simulink model "SAME5xPIM_MCLV2_MotorControl_Simulation"  (R2020b)
settings: Solver=ode45  StartTime=0.0  StopTime=10  FixedStep=0.001  MaxStep=1e-4  RelTol=1e-3  EnableMultiTasking=on
undefined symbols (not defined in the file or in its folder): DiscIntNeverNeededParam
libraries: simulink x8
Description:
  | Motor Control Simulation Demo
  | contacts : romain.delpoux@insa-lyon.fr, lubin.kerhuel@microchip.com
settings Model: DSRTSU_INTERNAL_RTI_VER=470  DSRTSU_INTERNAL_RTI_TYPE=rti1104  DSRTSU_INTERNAL_RTIFPGA=60  Creator=rdelpoux  LastModifiedBy=promu
settings SolverCC: ZeroCrossControl=DisableAll
settings DataIOCC: LimitDataPoints=on  SaveFormat=Array  ReturnWorkspaceOutputs=off
settings OptimizationCC: BlockReduction=off  OptimizeBlockIOStorage=off  BufferReuse=off  GlobalBufferReuse=off  ExpressionFolding=off  LocalBlockOutputs=off  LifeSpan=inf  OptimizeDataStoreBuffers=off  BusAssignmentInplaceUpdate=off
settings DebuggingCC: SolverPrmCheckMsg=warning  SFUnexpectedBacktrackingDiag=warning  SFNoUnconditionalDefaultTransitionDiag=warning  SFExecutionAtInitializationDiag=none  ArithmeticOperatorsInVariantConditions=warning
settings HardwareCC: ProdBitPerPointer=32  ProdBitPerSizeT=32  ProdBitPerPtrDiffT=32  ProdLargestAtomicInteger=Integer  ProdEndianess=BigEndian  ProdWordSize=32  ProdHWDeviceType=Generic->Custom  TargetIntDivRoundTo=Zero  TargetEndianess=BigEndian  TargetHWDeviceType=Generic->Custom
settings ModelReferenceCC: PropagateSignalLabelsOutOfModel=off
settings SFSimCC: SimUseLocalCustomCode=off  CustomCodeUndefinedFunction=UseInterfaceOnly
settings RTWCC: Description=dSPACE DS1104 Hardware Platform  SystemTargetFile=rti1104.tlc  MakeCommand=make_rti  TemplateMakefile=rti1104.tmf  RTWUseLocalCustomCode=off
settings CodeAppCC: StateflowObjectComments=on
settings STFCustomTargetCC: ParMdlRefBuildCompliant=on  ConcurrentExecutionCompliant=off  MatFileLogging=on  CPPClassGenCompliant=off  SystemTargetFile=rti1104.tlc
settings GRTTargetCC: TargetLangStandard=C89/C90 (ANSI)  CompOptLevelCompliant=off  ConcurrentExecutionCompliant=off  CombineOutputUpdateFcns=off  CPPClassGenCompliant=off  GRTInterface=on  UseToolchainInfoCompliant=off  ExtModeMexFile=noextcomm
settings ConfigComp: CovMetricSettings=dw  CovSaveCumulativeToWorkspaceVar=on  CovSaveSingleToWorkspaceVar=on  CovExternalEMLEnable=off  CovSFcnEnable=off

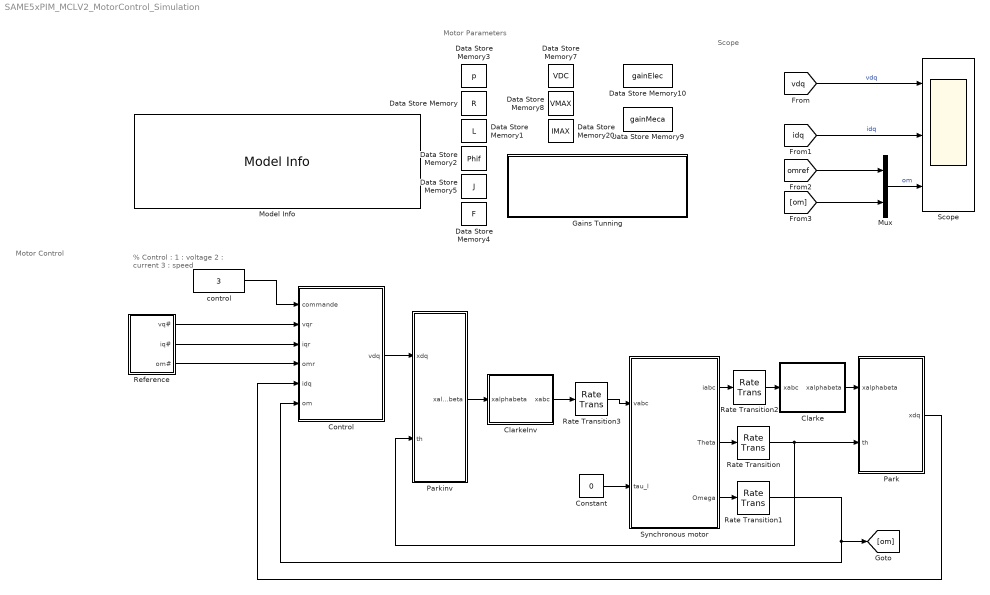
== system SAME5xPIM_MCLV2_MotorControl_Simulation ==
  note: Scope
  note: Motor Control
  note: % Control :
      | 1 : voltage
      | 2 : current
      | 3 : speed
  note: Motor Parameters
  Clarke : Subsystem
  ClarkeInv : Subsystem
  Constant : Constant  Value=0
  Control : Subsystem
  Data Store Memory : DataStoreMemory  DataStoreName=R  ReadBeforeWriteMsg=warning  WriteAfterWriteMsg=warning  WriteAfterReadMsg=warning  InitialValue=0.656  ShowAdditionalParam=off  OutDataTypeStr=single
  Data Store Memory1 : DataStoreMemory  DataStoreName=L  ReadBeforeWriteMsg=warning  WriteAfterWriteMsg=warning  WriteAfterReadMsg=warning  InitialValue=0.35e-3  ShowAdditionalParam=off  OutDataTypeStr=single
  Data Store Memory10 : DataStoreMemory  DataStoreName=gainElec  ReadBeforeWriteMsg=warning  WriteAfterWriteMsg=warning  WriteAfterReadMsg=warning  InitialValue=[0;0]  ShowAdditionalParam=off  OutDataTypeStr=single
  Data Store Memory2 : DataStoreMemory  DataStoreName=Phif  ReadBeforeWriteMsg=warning  WriteAfterWriteMsg=warning  WriteAfterReadMsg=warning  InitialValue=0.0066  ShowAdditionalParam=off  OutDataTypeStr=single
  Data Store Memory20 : DataStoreMemory  DataStoreName=IMAX  ReadBeforeWriteMsg=warning  WriteAfterWriteMsg=warning  WriteAfterReadMsg=warning  InitialValue=4  ShowAdditionalParam=off  OutDataTypeStr=int16
  Data Store Memory3 : DataStoreMemory  DataStoreName=p  ReadBeforeWriteMsg=warning  WriteAfterWriteMsg=warning  WriteAfterReadMsg=warning  InitialValue=4  ShowAdditionalParam=off  OutDataTypeStr=int16
  Data Store Memory4 : DataStoreMemory  DataStoreName=F  ReadBeforeWriteMsg=warning  WriteAfterWriteMsg=warning  WriteAfterReadMsg=warning  InitialValue=1.0e-05  ShowAdditionalParam=off  OutDataTypeStr=single
  Data Store Memory5 : DataStoreMemory  DataStoreName=J  ReadBeforeWriteMsg=warning  WriteAfterWriteMsg=warning  WriteAfterReadMsg=warning  InitialValue=1.0e-05  ShowAdditionalParam=off  OutDataTypeStr=single
  Data Store Memory7 : DataStoreMemory  DataStoreName=VDC  ReadBeforeWriteMsg=warning  WriteAfterWriteMsg=warning  WriteAfterReadMsg=warning  InitialValue=24  ShowAdditionalParam=off  OutMin=[-30]  OutMax=[30]  OutDataTypeStr=fixdt(1,16)
  Data Store Memory8 : DataStoreMemory  DataStoreName=VMAX  ReadBeforeWriteMsg=warning  WriteAfterWriteMsg=warning  WriteAfterReadMsg=warning  InitialValue=12  ShowAdditionalParam=off  OutMin=[-30]  OutMax=[30]  OutDataTypeStr=fixdt(1,16)
  Data Store Memory9 : DataStoreMemory  DataStoreName=gainMeca  ReadBeforeWriteMsg=warning  WriteAfterWriteMsg=warning  WriteAfterReadMsg=warning  InitialValue=[0;0]  ShowAdditionalParam=off  OutDataTypeStr=single
  Gains Tunning : Subsystem
  Model Info : simulink/Model-Wide Utilities/Model Info  Frame=on  DisplayStringWithTags=|  HorizontalTextAlignment=Center  LeftAlignmentValue=0.5
      | %<ModelName> v%<ModelVersion> - %<Creator>
      | 
      | %<Description>
      | 
      | Last modified on: %<LastModificationDate>
  Mux : Mux  Inputs=2
  "Park " : Subsystem
  Parkinv : Subsystem
  Rate Transition{,1..3} (4 alike) : RateTransition  OutPortSampleTime=1e-4
  Reference : Subsystem
  Scope : Scope  NumInputPorts=3
  Synchronous motor : Subsystem  mask(Test){Rmodel=0.656, Lmodel=0.35e-3, Phifmodel=0.0066, pmodel=4, Jmodel=1.e-05, fmodel=1.e-05, C0Model=0.01}
      mask prompts: Rmodel "Phase resistor R (Ohm)"; Lmodel "Phase Inductor L (H)"; Phifmodel "Rotor flux Phif (Wb)"; pmodel "Pole paires"; Jmodel "Inertia J (kg.m^2)"; fmodel "Fluide friction f (N.m.s/rad)"; C0Model "Dry friction C0 (N.m)"
      mask Help: disp('{\itEquation:}  \alpha^2 + \beta^2 \rightarrow \gamma^2, \chi, \phi_3 = {\bfcool}', 'texmode','on')
      mask DialogControl DescGroupVar Prompt: PMSM
      mask DialogControl DescTextVar Prompt: Motor Model
      mask DialogControl Container3 Prompt: Electrical parameters
      mask DialogControl Container4 Prompt: Mechanical parameter
  control : Constant  Value=3
  wires:
  Parkinv/1(xalphabeta) -> ClarkeInv/1(xalphabeta)
  ClarkeInv/1(xabc) -> Rate Transition3/1
  Rate Transition2/1 -> Clarke/1(xabc)
  Clarke/1(xalphabeta) -> "Park "/1(xalphabeta)
  "Park "/1(xdq) -> Control/5(idq)
  Reference/2(iq#) -> Control/3(iqr)
  Rate Transition1/1 -> [om], Control/6(om)
  Reference/3(om#) -> Control/4(omr)
  Rate Transition/1 -> Parkinv/2(th), "Park "/2(th)
  Control/1(vdq) -> Parkinv/1(xdq)
  Synchronous motor/3(Omega) -> Rate Transition1/1
  Synchronous motor/2(Theta) -> Rate Transition/1
  Synchronous motor/1(iabc) -> Rate Transition2/1
  Rate Transition3/1 -> Synchronous motor/1(vabc)
  control/1 -> Control/1(commande)
  Constant/1 -> Synchronous motor/2(tau_l)
  Reference/1(vq#) -> Control/2(vqr)
  [vdq] -> Scope/1  "vdq"
  [idq] -> Scope/2  "idq"
  [omref] -> Mux/1
  [om] -> Mux/2
  Mux/1 -> Scope/3  "om"

== system SAME5xPIM_MCLV2_MotorControl_Simulation/Clarke ==
  note: Clarke inverse
  xabc : Inport
  C23 : Gain  Gain=|  Multiplication=Matrix(K*u)
      | [1   -1/2        -1/2;
      |         0   sqrt(3)/2   -sqrt(3)/2]
  Gain : Gain  Gain=2/3
  xalphabeta : Outport  VectorParamsAs1DForOutWhenUnconnected=off
  wires:
  Gain/1 -> C23/1
  C23/1 -> xalphabeta/1
  xabc/1 -> Gain/1

== system SAME5xPIM_MCLV2_MotorControl_Simulation/ClarkeInv ==
  note: Clarke inverse
  xalphabeta : Inport
  C23' : Gain  Gain=|  Multiplication=Matrix(K*u)
      | [1   -1/2        -1/2;
      |         0   sqrt(3)/2   -sqrt(3)/2]'
  xabc : Outport  VectorParamsAs1DForOutWhenUnconnected=off
  wires:
  C23'/1 -> xabc/1
  xalphabeta/1 -> C23'/1

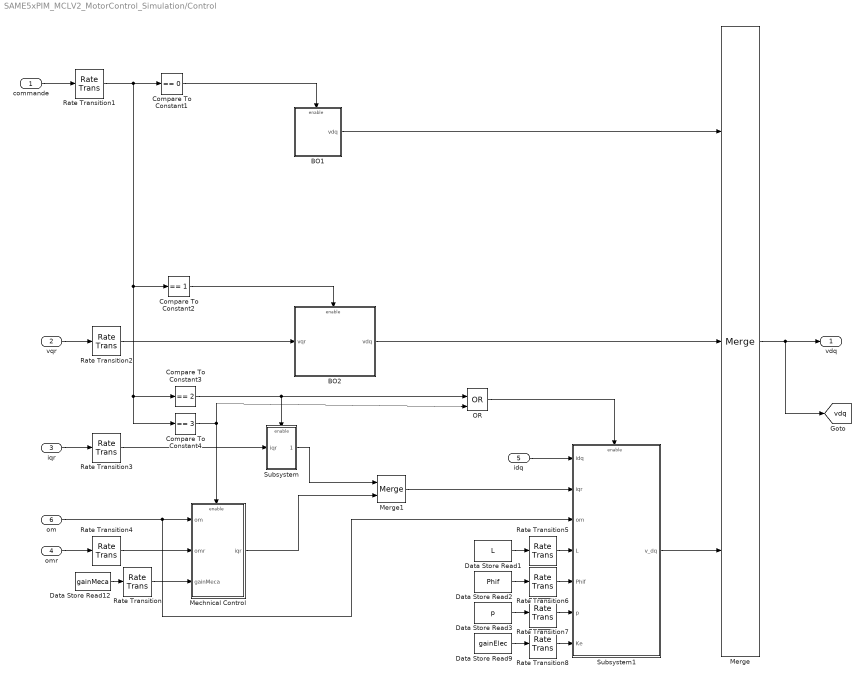
== system SAME5xPIM_MCLV2_MotorControl_Simulation/Control ==
  commande : Inport
  vqr : Inport  Port=2
  iqr : Inport  Port=3
  omr : Inport  Port=4
  idq : Inport  Port=5
  om : Inport  Port=6
  BO1 : Subsystem
  BO2 : Subsystem
  Compare To Constant1 : simulink/Logic and Bit Operations/Compare To Constant  relop===  const=0  OutDataTypeStr=boolean
  Compare To Constant2 : simulink/Logic and Bit Operations/Compare To Constant  relop===  const=1  OutDataTypeStr=boolean
  Compare To Constant3 : simulink/Logic and Bit Operations/Compare To Constant  relop===  const=2  OutDataTypeStr=boolean
  Compare To Constant4 : simulink/Logic and Bit Operations/Compare To Constant  relop===  const=3  OutDataTypeStr=boolean
  Data Store Read1 : DataStoreRead  DataStoreName=L  SampleTime=1
  Data Store Read12 : DataStoreRead  DataStoreName=gainMeca  SampleTime=1
  Data Store Read2 : DataStoreRead  DataStoreName=Phif  SampleTime=1
  Data Store Read3 : DataStoreRead  DataStoreName=p  SampleTime=1
  Data Store Read9 : DataStoreRead  DataStoreName=gainElec  SampleTime=1
  Mechnical Control : Subsystem
  Merge : Merge  Inputs=3
  Merge1 : Merge
  OR : Logic  Operator=OR  IconShape=distinctive  AllPortsSameDT=off  OutDataTypeStr=boolean
  Rate Transition{,1..8} (9 alike) : RateTransition
  Subsystem : Subsystem
  Subsystem1 : Subsystem
  vdq : Outport  VectorParamsAs1DForOutWhenUnconnected=off
  tag scope: vdq=global
  wires:
  Rate Transition8/1 -> Subsystem1/7(Ke)
  Rate Transition7/1 -> Subsystem1/6(p)
  Rate Transition6/1 -> Subsystem1/5(Phif)
  Rate Transition5/1 -> Subsystem1/4(L)
  Rate Transition/1 -> Mechnical Control/3(gainMeca)
  Rate Transition4/1 -> Mechnical Control/2(omr)
  Rate Transition3/1 -> Subsystem/1(iqr)
  Rate Transition2/1 -> BO2/1(vqr)
  Subsystem1/1(v_dq) -> Merge/3
  Merge1/1 -> Subsystem1/2(iqr)
  idq/1 -> Subsystem1/1(idq)
  OR/1 -> Subsystem1/Enable
  om/1 -> Mechnical Control/1(om), Subsystem1/3(om)
  Compare To Constant4/1 -> Mechnical Control/Enable, OR/2
  Mechnical Control/1(iqr) -> Merge1/2
  Subsystem/1(Out1) -> Merge1/1
  Rate Transition1/1 -> Compare To Constant1/1, Compare To Constant4/1, Compare To Constant3/1, Compare To Constant2/1
  Compare To Constant3/1 -> Subsystem/Enable, OR/1
  Compare To Constant1/1 -> BO1/Enable
  commande/1 -> Rate Transition1/1
  Merge/1 -> [vdq], vdq/1
  Compare To Constant2/1 -> BO2/Enable
  BO1/1(vdq) -> Merge/1
  BO2/1(vdq) -> Merge/2
  Data Store Read9/1 -> Rate Transition8/1
  Data Store Read1/1 -> Rate Transition5/1
  Data Store Read3/1 -> Rate Transition7/1
  Data Store Read2/1 -> Rate Transition6/1
  vqr/1 -> Rate Transition2/1
  iqr/1 -> Rate Transition3/1
  omr/1 -> Rate Transition4/1
  Data Store Read12/1 -> Rate Transition/1

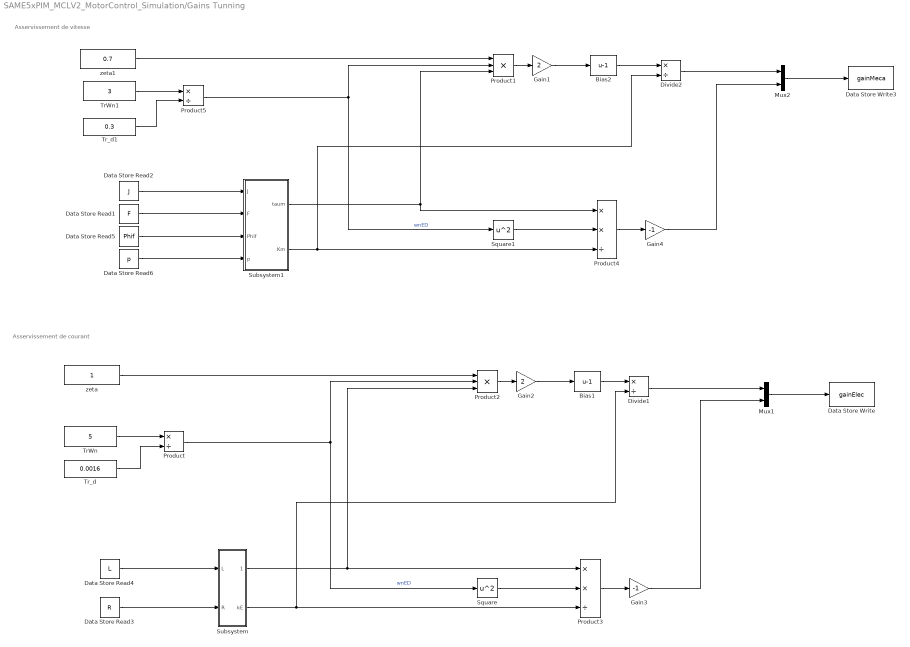
== system SAME5xPIM_MCLV2_MotorControl_Simulation/Gains Tunning ==
  note: Asservissement de courant
  note: Asservissement de vitesse
  Bias1 : Bias  Bias=-1
  Bias2 : Bias  Bias=-1
  Data Store Read1 : DataStoreRead  DataStoreName=F  SampleTime=1
  Data Store Read2 : DataStoreRead  DataStoreName=J  SampleTime=1
  Data Store Read3 : DataStoreRead  DataStoreName=R  SampleTime=1
  Data Store Read4 : DataStoreRead  DataStoreName=L  SampleTime=1
  Data Store Read5 : DataStoreRead  DataStoreName=Phif  SampleTime=1
  Data Store Read6 : DataStoreRead  DataStoreName=p  SampleTime=1
  Data Store Write : DataStoreWrite  DataStoreName=gainElec  SampleTime=1
  Data Store Write3 : DataStoreWrite  DataStoreName=gainMeca
  Divide1 : Product  Inputs=*/
  Divide2 : Product  Inputs=*/
  Gain1 : Gain  Gain=2
  Gain2 : Gain  Gain=2
  Gain3 : Gain  Gain=-1
  Gain4 : Gain  Gain=-1
  Mux1 : Mux  Inputs=2
  Mux2 : Mux  Inputs=2
  Product : Product  Inputs=*/
  Product1 : Product  Inputs=3
  Product2 : Product  Inputs=3
  Product3 : Product  Inputs=**/
  Product4 : Product  Inputs=**/
  Product5 : Product  Inputs=*/
  Square : Math  Operator=square  SaturateOnIntegerOverflow=on
  Square1 : Math  Operator=square  SaturateOnIntegerOverflow=on
  Subsystem : Subsystem
  Subsystem1 : Subsystem
  TrWn : Constant  Value=5  OutDataTypeStr=single
  TrWn1 : Constant  Value=3  OutDataTypeStr=single
  Tr_d : Constant  Value=0.0016  OutDataTypeStr=single
  Tr_d1 : Constant  Value=0.3  OutDataTypeStr=single
  zeta : Constant  OutDataTypeStr=single
  zeta1 : Constant  Value=0.7  OutDataTypeStr=single
  wires:
  Gain3/1 -> Mux1/2
  Product3/1 -> Gain3/1
  Divide1/1 -> Mux1/1
  Bias1/1 -> Divide1/1
  Product2/1 -> Gain2/1
  Mux1/1 -> Data Store Write/1
  Data Store Read4/1 -> Subsystem/1(L)
  Data Store Read3/1 -> Subsystem/2(R)
  Subsystem/1(tauE) -> Product2/3, Product3/1
  TrWn/1 -> Product/1
  Tr_d/1 -> Product/2
  Product/1 -> Product2/2, Square/1  "wnED"
  Subsystem/2(kE) -> Divide1/2, Product3/3
  Gain2/1 -> Bias1/1
  zeta/1 -> Product2/1
  Square/1 -> Product3/2
  Square1/1 -> Product4/2
  Gain1/1 -> Bias2/1
  Product1/1 -> Gain1/1
  Bias2/1 -> Divide2/1
  Divide2/1 -> Mux2/1
  Product4/1 -> Gain4/1
  Gain4/1 -> Mux2/2
  Mux2/1 -> Data Store Write3/1
  Data Store Read2/1 -> Subsystem1/1(J)
  Data Store Read1/1 -> Subsystem1/2(F)
  Data Store Read5/1 -> Subsystem1/3(Phif)
  Data Store Read6/1 -> Subsystem1/4(p)
  Tr_d1/1 -> Product5/2
  TrWn1/1 -> Product5/1
  zeta1/1 -> Product1/1
  Product5/1 -> Square1/1, Product1/2  "wnED"
  Subsystem1/1(taum) -> Product4/1, Product1/3
  Subsystem1/2(Km) -> Divide2/2, Product4/3

== system SAME5xPIM_MCLV2_MotorControl_Simulation/Park  ==
  note: Inverse Park
  xalphabeta : Inport
  th : Inport  Port=2
  Fcn : Fcn  Expr=u(1)*cos(4*u(3))+u(2)*sin(4*u(3))
  Fcn1 : Fcn  Expr=-u(1)*sin(4*u(3))+u(2)*cos(4*u(3))
  Mux : Mux  Inputs=2
  Mux1 : Mux  Inputs=2
  xdq : Outport  VectorParamsAs1DForOutWhenUnconnected=off
  tag scope: idq=global
  wires:
  xalphabeta/1 -> Mux/1
  th/1 -> Mux/2
  Mux/1 -> Fcn1/1, Fcn/1
  Fcn/1 -> Mux1/1
  Fcn1/1 -> Mux1/2
  Mux1/1 -> [idq], xdq/1

== system SAME5xPIM_MCLV2_MotorControl_Simulation/Parkinv ==
  note: Inverse Park
  xdq : Inport
  th : Inport  Port=2
  Fcn : Fcn  Expr=u(1)*cos(4*u(3))-u(2)*sin(4*u(3))
  Fcn1 : Fcn  Expr=u(1)*sin(4*u(3))+u(2)*cos(4*u(3))
  Mux : Mux  Inputs=2
  Mux1 : Mux  Inputs=2
  xalphabeta : Outport  VectorParamsAs1DForOutWhenUnconnected=off
  wires:
  Mux1/1 -> xalphabeta/1
  Fcn1/1 -> Mux1/2
  Fcn/1 -> Mux1/1
  Mux/1 -> Fcn/1, Fcn1/1
  th/1 -> Mux/2
  xdq/1 -> Mux/1

== system SAME5xPIM_MCLV2_MotorControl_Simulation/Reference ==
  Step : Step  Time=2  After=2  OutDataTypeStr=single  SampleTime=0
  Step1 : Step  Time=2  After=300  OutDataTypeStr=single  SampleTime=0
  Step2 : Step  Time=2  After=5  OutDataTypeStr=single  SampleTime=0
  vq# : Outport  VectorParamsAs1DForOutWhenUnconnected=off
  iq# : Outport  Port=2  VectorParamsAs1DForOutWhenUnconnected=off
  om# : Outport  Port=3  VectorParamsAs1DForOutWhenUnconnected=off
  tag scope: omref=global
  wires:
  Step/1 -> iq#/1
  Step1/1 -> [omref], om#/1
  Step2/1 -> vq#/1

== system SAME5xPIM_MCLV2_MotorControl_Simulation/Synchronous motor ==
  vabc : Inport
  tau_l : Inport  Port=2
  Data Type Conversion : DataTypeConversion  OutDataTypeStr=single
  Data Type Conversion1 : DataTypeConversion  OutDataTypeStr=single
  Data Type Conversion2 : DataTypeConversion  OutDataTypeStr=single
  Electrique : Subsystem
  Mécanique : Subsystem
  iabc : Outport  VectorParamsAs1DForOutWhenUnconnected=off
  Theta : Outport  Port=2  VectorParamsAs1DForOutWhenUnconnected=off
  Omega : Outport  Port=3  VectorParamsAs1DForOutWhenUnconnected=off
  wires:
  vabc/1 -> Electrique/1(vabc)
  tau_l/1 -> Mécanique/2(tau_l)
  Electrique/1(iabc) -> Data Type Conversion/1
  Mécanique/1(Theta) -> Electrique/3(Theta), Data Type Conversion1/1
  Mécanique/2(Omega) -> Electrique/2(Omega), Data Type Conversion2/1
  Electrique/2(tau_m) -> Mécanique/1(tau_m)
  Data Type Conversion/1 -> iabc/1
  Data Type Conversion1/1 -> Theta/1
  Data Type Conversion2/1 -> Omega/1

== system SAME5xPIM_MCLV2_MotorControl_Simulation/Control/BO1 ==
  Enable : EnablePort
  Mux : Mux  Inputs=2
  vd : Constant  Value=0  OutMin=[-12]  OutMax=[12]  OutDataTypeStr=single
  vq : Constant  Value=0  OutMin=[-12]  OutMax=[12]  OutDataTypeStr=single
  vdq : Outport  VectorParamsAs1DForOutWhenUnconnected=off
  wires:
  vd/1 -> Mux/1
  Mux/1 -> vdq/1
  vq/1 -> Mux/2

== system SAME5xPIM_MCLV2_MotorControl_Simulation/Control/BO2 ==
  vqr : Inport
  Enable : EnablePort
  Constant : Constant  Value=0  OutDataTypeStr=single
  Mux : Mux  Inputs=2
  vdq : Outport  VectorParamsAs1DForOutWhenUnconnected=off
  wires:
  vqr/1 -> Mux/2
  Constant/1 -> Mux/1
  Mux/1 -> vdq/1

== system SAME5xPIM_MCLV2_MotorControl_Simulation/Control/Mechnical Control ==
  om : Inport
  omr : Inport  Port=2
  gainMeca : Inport  Port=3
  Enable : EnablePort  StatesWhenEnabling=reset
  Augmented state feedback : Subsystem
      settings: PortSchema="{\"entries\":[{\"content\":{\"sides\":[{\"content\":{\"connectorIds\":[\"In1\",\"In2\"]},\"type\":\"ConnectorPlacement.EquallySpacedRectSide\",\"uuid\":\"89137e2f-cd18-4dcc-a524-9caf5367be1f\"},{\"content\":{\"connectorIds\":[\"Out1\"],\"side\":\"RIGHT\"},\"type\":\"ConnectorPlacement.EquallySpacedRectSide\",\"uuid\":\"4fa0fb61-d5d6-47b2-9e74-7b8a54a26f7d\"},{\"content\":{\"connectorIds\":[],\"side\":\"TOP\"},\"type\":\"ConnectorPlacement.EquallySpacedRectSide\",\"uuid\":\"143a26d0-3cb3-43f1-872c-87316c90bc9f\"},{\"content\":{\"connectorIds\":[\"In3\"],\"side\":\"BOTTOM\"},\"type\":\"ConnectorPlacement.EquallySpacedRectSide\",\"uuid\":\"8516086b-4f00-45b1-b860-126256ccf69b\"},{\"content\":{\"connectorIds\":[],\"side\":\"HIDDEN\"},\"type\":\"ConnectorPlacement.EquallySpacedRectSide\",\"uuid\":\"abbfb321-16c4-4def-9c9f-eddb440e6971\"}]},\"type\":\"ConnectorPlacement.EquallySpacedConnector\",\"uuid\":\"ad3527e6-0bb9-4e51-b689-1365c7b23b5d\"}],\"packageUris\":[\"http://schema.mathworks.com/mf0/Connector/R2020b\"],\"version\":\"1.0\"}"
  iqr : Outport  VectorParamsAs1DForOutWhenUnconnected=off
  wires:
  om/1 -> Augmented state feedback/2(om)
  Augmented state feedback/1(iqref) -> iqr/1
  omr/1 -> Augmented state feedback/1(omref)
  gainMeca/1 -> Augmented state feedback/3(gainMeca)

== system SAME5xPIM_MCLV2_MotorControl_Simulation/Control/Subsystem ==
  iqr : Inport
  Enable : EnablePort
  Out1 : Outport
  wires:
  iqr/1 -> Out1/1

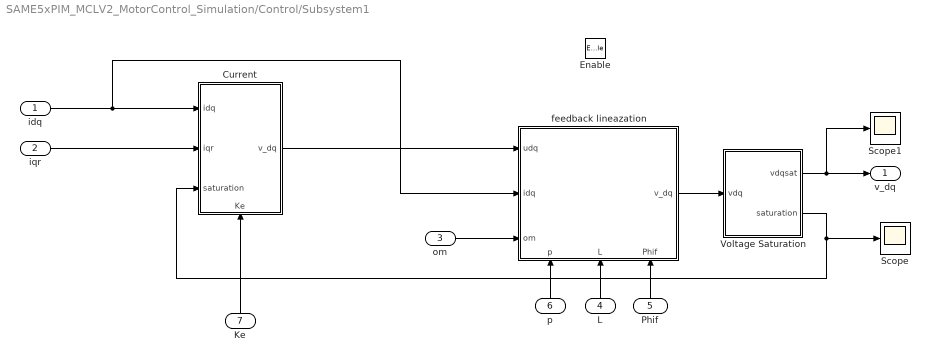
== system SAME5xPIM_MCLV2_MotorControl_Simulation/Control/Subsystem1 ==
  idq : Inport
  iqr : Inport  Port=2
  om : Inport  Port=3
  L : Inport  Port=4
  Phif : Inport  Port=5
  p : Inport  Port=6
  Ke : Inport  Port=7
  Enable : EnablePort  StatesWhenEnabling=reset
  Current : Subsystem
      settings: PortSchema="{\"entries\":[{\"content\":{\"sides\":[{\"content\":{\"connectorIds\":[\"In1\",\"In2\",\"In3\"]},\"type\":\"ConnectorPlacement.EquallySpacedRectSide\",\"uuid\":\"0dd1bd5c-4f2d-4a51-9bc2-8bf74640d4ff\"},{\"content\":{\"connectorIds\":[\"Out1\"],\"side\":\"RIGHT\"},\"type\":\"ConnectorPlacement.EquallySpacedRectSide\",\"uuid\":\"9ff54608-efe8-47a2-97c0-1c2807ae0451\"},{\"content\":{\"connectorIds\":[],\"side\":\"TOP\"},\"type\":\"ConnectorPlacement.EquallySpacedRectSide\",\"uuid\":\"a5b0a1bc-2629-443b-a6ad-4c332df72e2c\"},{\"content\":{\"connectorIds\":[\"In4\"],\"side\":\"BOTTOM\"},\"type\":\"ConnectorPlacement.EquallySpacedRectSide\",\"uuid\":\"e8d63822-9705-4716-821c-9412f2966827\"},{\"content\":{\"connectorIds\":[],\"side\":\"HIDDEN\"},\"type\":\"ConnectorPlacement.EquallySpacedRectSide\",\"uuid\":\"63401b5c-75e9-49e9-aa08-12658d9987d3\"}]},\"type\":\"ConnectorPlacement.EquallySpacedConnector\",\"uuid\":\"d3f45542-3ea7-483a-a2ee-6c72d9ae8820\"}],\"packageUris\":[\"http://schema.mathworks.com/mf0/Connector/R2020b\"],\"version\":\"1.0\"}"
  Scope : Scope
  Scope1 : Scope
  Voltage Saturation : Subsystem
  feedback lineazation : Subsystem
      settings: PortSchema="{\"entries\":[{\"content\":{\"sides\":[{\"content\":{\"connectorIds\":[\"In1\",\"In2\",\"In3\"]},\"type\":\"ConnectorPlacement.EquallySpacedRectSide\",\"uuid\":\"169b5321-ee7c-423e-8449-192a786c9798\"},{\"content\":{\"connectorIds\":[\"Out1\"],\"side\":\"RIGHT\"},\"type\":\"ConnectorPlacement.EquallySpacedRectSide\",\"uuid\":\"910fdd05-0903-4759-8f85-a6669ffcf15d\"},{\"content\":{\"connectorIds\":[],\"side\":\"TOP\"},\"type\":\"ConnectorPlacement.EquallySpacedRectSide\",\"uuid\":\"8e0cf6ac-18cd-4e02-9312-1598b8dbe459\"},{\"content\":{\"connectorIds\":[\"In4\",\"In5\",\"In6\"],\"side\":\"BOTTOM\"},\"type\":\"ConnectorPlacement.EquallySpacedRectSide\",\"uuid\":\"bf7c0436-036d-4f64-97d8-e9b131650054\"},{\"content\":{\"connectorIds\":[],\"side\":\"HIDDEN\"},\"type\":\"ConnectorPlacement.EquallySpacedRectSide\",\"uuid\":\"cd87405f-25ee-425b-a181-6989070156fa\"}]},\"type\":\"ConnectorPlacement.EquallySpacedConnector\",\"uuid\":\"912b1b6f-c896-42c8-9325-248c15d73689\"}],\"packageUris\":[\"http://schema.mathworks.com/mf0/Connector/R2020b\"],\"version\":\"1.0\"}"
  v_dq : Outport
  wires:
  om/1 -> feedback lineazation/3(om)
  L/1 -> feedback lineazation/5(L)
  Phif/1 -> feedback lineazation/6(Phif)
  p/1 -> feedback lineazation/4(p)
  Voltage Saturation/1(vdqsat) -> Scope1/1, v_dq/1
  iqr/1 -> Current/2(iqr)
  Current/1(v_dq) -> feedback lineazation/1(udq)
  idq/1 -> feedback lineazation/2(idq), Current/1(idq)
  Ke/1 -> Current/4(Ke)
  Voltage Saturation/2(saturation) -> Scope/1, Current/3(saturation)
  feedback lineazation/1(v_dq) -> Voltage Saturation/1(vdq)

== system SAME5xPIM_MCLV2_MotorControl_Simulation/Gains Tunning/Subsystem ==
  L : Inport
  R : Inport  Port=2
  Divide1 : Product  Inputs=/
  Divide2 : Product  Inputs=*/
  tauE : Outport
  kE : Outport  Port=2
  wires:
  Divide2/1 -> tauE/1  "tauE"
  R/1 -> Divide1/1, Divide2/2
  L/1 -> Divide2/1
  Divide1/1 -> kE/1  "kE"

== system SAME5xPIM_MCLV2_MotorControl_Simulation/Gains Tunning/Subsystem1 ==
  J : Inport
  F : Inport  Port=2
  Phif : Inport  Port=3
  p : Inport  Port=4
  Divide3 : Product  Inputs=*/
  Divide6 : Product  Inputs=*/
  Divide7 : Product  Inputs=**
  Gain : Gain  Gain=3/2
  taum : Outport
  Km : Outport  Port=2
  wires:
  Gain/1 -> Divide7/1
  F/1 -> Divide3/2, Divide6/2
  J/1 -> Divide6/1
  p/1 -> Divide7/2
  Divide3/1 -> Km/1  "Km"
  Phif/1 -> Gain/1
  Divide6/1 -> taum/1  "taum"
  Divide7/1 -> Divide3/1  "Km"

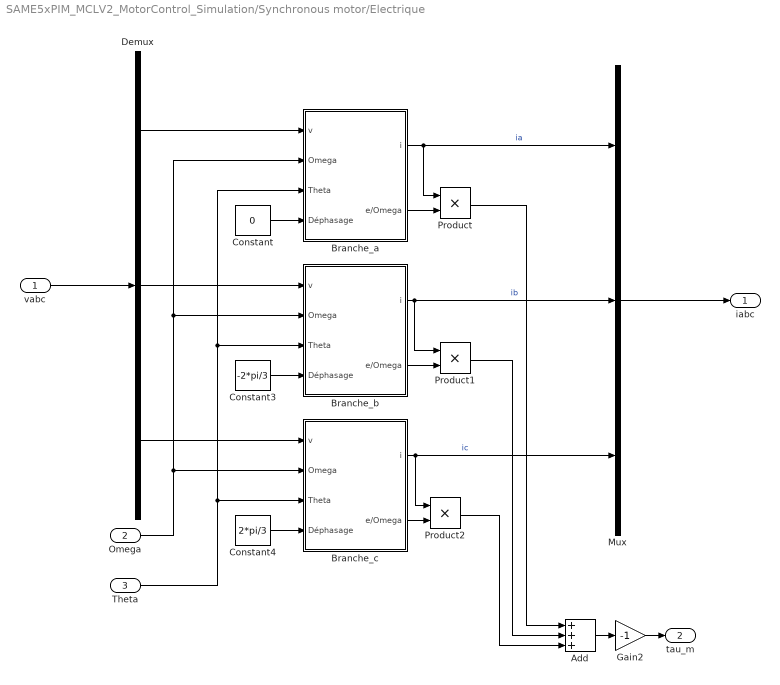
== system SAME5xPIM_MCLV2_MotorControl_Simulation/Synchronous motor/Electrique ==
  vabc : Inport
  Omega : Inport  Port=2
  Theta : Inport  Port=3
  Add : Sum  Inputs=+++
  Branche_a : Subsystem
  Branche_b : Subsystem
  Branche_c : Subsystem
  Constant : Constant  Value=0
  Constant3 : Constant  Value=-2*pi/3
  Constant4 : Constant  Value=2*pi/3
  Demux : Demux  Outputs=3
  Gain2 : Gain  Gain=-1
  Mux : Mux  Inputs=3
  Product : Product
  Product1 : Product
  Product2 : Product
  iabc : Outport  VectorParamsAs1DForOutWhenUnconnected=off
  tau_m : Outport  Port=2  VectorParamsAs1DForOutWhenUnconnected=off
  wires:
  Branche_c/1(i) -> Product2/1, Mux/3  "ic"
  Demux/1 -> Branche_a/1(v)
  Demux/2 -> Branche_b/1(v)
  Constant/1 -> Branche_a/4(Déphasage)
  Constant3/1 -> Branche_b/4(Déphasage)
  Constant4/1 -> Branche_c/4(Déphasage)
  Branche_b/1(i) -> Mux/2, Product1/1  "ib"
  Branche_a/1(i) -> Mux/1, Product/1  "ia"
  Demux/3 -> Branche_c/1(v)
  Theta/1 -> Branche_a/3(Theta), Branche_b/3(Theta), Branche_c/3(Theta)
  Omega/1 -> Branche_a/2(Omega), Branche_b/2(Omega), Branche_c/2(Omega)
  Branche_a/2(e/Omega) -> Product/2
  Branche_b/2(e/Omega) -> Product1/2
  Branche_c/2(e/Omega) -> Product2/2
  Product2/1 -> Add/3
  Product1/1 -> Add/2
  Product/1 -> Add/1
  Add/1 -> Gain2/1
  Gain2/1 -> tau_m/1
  Mux/1 -> iabc/1
  vabc/1 -> Demux/1

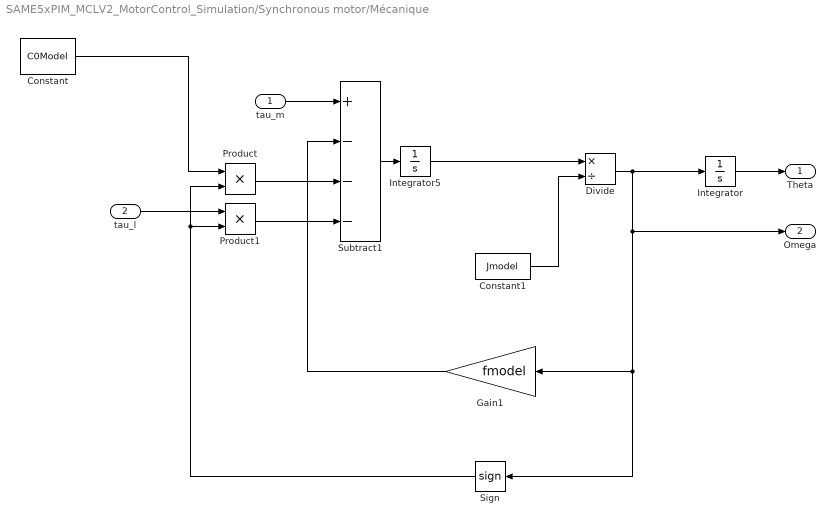
== system SAME5xPIM_MCLV2_MotorControl_Simulation/Synchronous motor/Mécanique ==
  tau_m : Inport
  tau_l : Inport  Port=2
  Constant : Constant  Value=C0Model
  Constant1 : Constant  Value=Jmodel
  Divide : Product  Inputs=*/
  Gain1 : Gain  Gain=fmodel
  Integrator : Integrator
  Integrator5 : Integrator
  Product : Product
  Product1 : Product
  Sign : Signum  ZeroCross=off
  Subtract1 : Sum  Inputs=+---
  Theta : Outport  VectorParamsAs1DForOutWhenUnconnected=off
  Omega : Outport  Port=2  VectorParamsAs1DForOutWhenUnconnected=off
  wires:
  Product/1 -> Subtract1/3
  Sign/1 -> Product1/2, Product/2
  Constant1/1 -> Divide/2
  Constant/1 -> Product/1
  tau_m/1 -> Subtract1/1
  Gain1/1 -> Subtract1/2
  Divide/1 -> Integrator/1, Omega/1, Gain1/1, Sign/1
  Integrator5/1 -> Divide/1
  tau_l/1 -> Product1/1
  Integrator/1 -> Theta/1
  Subtract1/1 -> Integrator5/1
  Product1/1 -> Subtract1/4

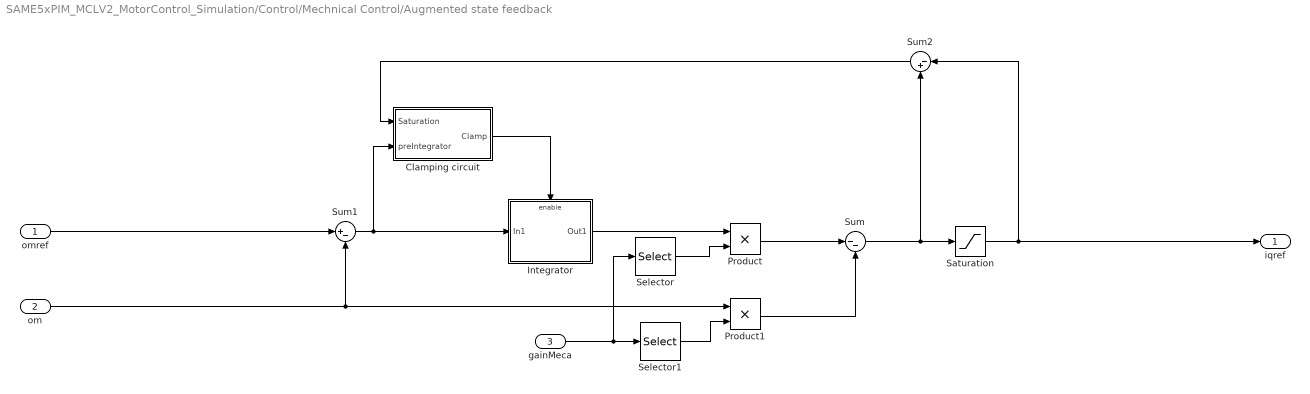
== system SAME5xPIM_MCLV2_MotorControl_Simulation/Control/Mechnical Control/Augmented state feedback ==
  omref : Inport
  om : Inport  Port=2
  gainMeca : Inport  Port=3
  Clamping circuit : Subsystem
  Integrator : Subsystem
  Product : Product
  Product1 : Product
  Saturation : Saturate  UpperLimit=4  LowerLimit=-4
  Selector : Selector  InputPortWidth=2  IndexOptions=Index vector (dialog)  Indices=[2]  OutputSizes=1
  Selector1 : Selector  InputPortWidth=2  IndexOptions=Index vector (dialog)  Indices=1  OutputSizes=1
  Sum : Sum  Inputs=|--  OutDataTypeStr=single  SaturateOnIntegerOverflow=on
  Sum1 : Sum  Inputs=|+-
  Sum2 : Sum  Inputs=|-+  OutDataTypeStr=Inherit: Same as accumulator  SaturateOnIntegerOverflow=on
  iqref : Outport  VectorParamsAs1DForOutWhenUnconnected=off
  wires:
  Sum/1 -> Sum2/2, Saturation/1
  Product1/1 -> Sum/2
  Product/1 -> Sum/1
  om/1 -> Sum1/2, Product1/1
  Sum1/1 -> Integrator/1(In1), Clamping circuit/2(preIntegrator)
  omref/1 -> Sum1/1
  Clamping circuit/1(Clamp) -> Integrator/Enable
  Sum2/1 -> Clamping circuit/1(Saturation)
  Integrator/1(Out1) -> Product/1
  Saturation/1 -> Sum2/1, iqref/1
  Selector1/1 -> Product1/2
  Selector/1 -> Product/2
  gainMeca/1 -> Selector1/1, Selector/1

== system SAME5xPIM_MCLV2_MotorControl_Simulation/Control/Subsystem1/Current ==
  idq : Inport
  iqr : Inport  Port=2
  saturation : Inport  Port=3
  Ke : Inport  Port=4
  Constant : Constant  Value=0
  Delay : Delay  DelayLength=1
  Gain1 : Gain  Gain=[1 0]  Multiplication=Matrix(K*u)  OutDataTypeStr=Inherit: Same as input
  Gain2 : Gain  Gain=[0 1]  Multiplication=Matrix(K*u)  OutDataTypeStr=Inherit: Same as input
  Gain3 : Gain  Gain=[1 0]  Multiplication=Matrix(K*u)  OutDataTypeStr=Inherit: Same as input
  Gain4 : Gain  Gain=[0 1]  Multiplication=Matrix(K*u)  OutDataTypeStr=Inherit: Same as input
  Mux1 : Mux  Inputs=2
  Subsystem1 : Subsystem
  Subsystem2 : Subsystem
  v_dq : Outport  VectorParamsAs1DForOutWhenUnconnected=off
  wires:
  Constant/1 -> Subsystem1/1(iref)
  saturation/1 -> Delay/1
  Subsystem2/1(v) -> Mux1/2
  Subsystem1/1(v) -> Mux1/1
  idq/1 -> Gain2/1, Gain1/1
  Gain1/1 -> Subsystem1/2(i)
  Gain2/1 -> Subsystem2/2(i)
  Mux1/1 -> v_dq/1
  Ke/1 -> Subsystem1/4(K_e), Subsystem2/4(K_e)
  Delay/1 -> Gain3/1, Gain4/1
  Gain3/1 -> Subsystem1/3(saturation)
  Gain4/1 -> Subsystem2/3(saturation)
  iqr/1 -> Subsystem2/1(iref)

== system SAME5xPIM_MCLV2_MotorControl_Simulation/Control/Subsystem1/Voltage Saturation ==
  vdq : Inport
  Divide : Product  Inputs=*/
  Gain : Gain  Gain=12
  Norm L2 : Subsystem
  Sum : Sum  Inputs=|+-
  Switch : Switch  Criteria=u2 > Threshold  Threshold=12
  vdqsat : Outport  VectorParamsAs1DForOutWhenUnconnected=off
  saturation : Outport  Port=2  VectorParamsAs1DForOutWhenUnconnected=off
  wires:
  Sum/1 -> saturation/1
  vdq/1 -> Switch/3, Sum/1, Divide/1, Norm L2/1(In1)
  Switch/1 -> vdqsat/1, Sum/2
  Divide/1 -> Gain/1
  Norm L2/1(y) -> Switch/2, Divide/2
  Gain/1 -> Switch/1

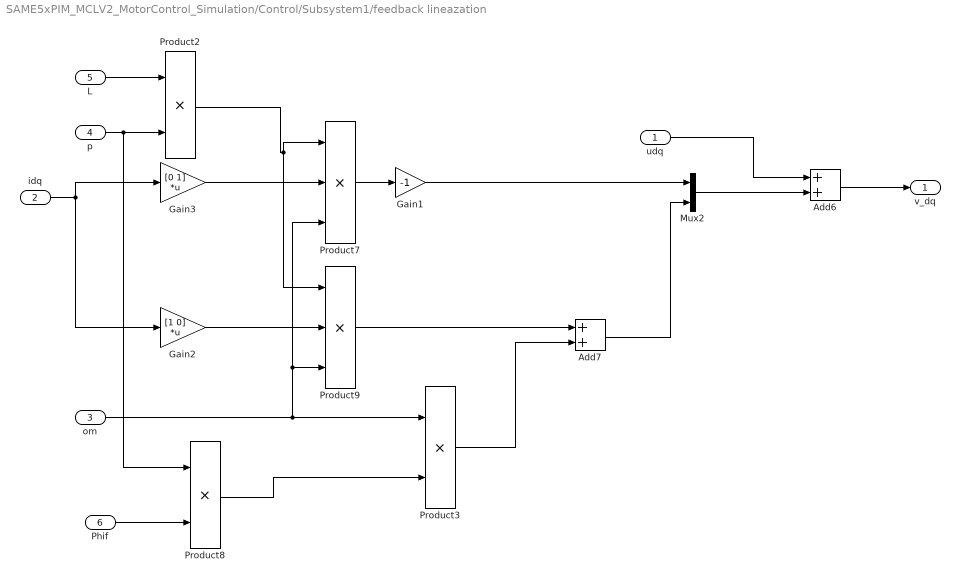
== system SAME5xPIM_MCLV2_MotorControl_Simulation/Control/Subsystem1/feedback lineazation ==
  udq : Inport
  idq : Inport  Port=2
  om : Inport  Port=3
  p : Inport  Port=4
  L : Inport  Port=5
  Phif : Inport  Port=6
  Add6 : Sum
  Add7 : Sum
  Gain1 : Gain  Gain=-1
  Gain2 : Gain  Gain=[1 0]  Multiplication=Matrix(K*u)
  Gain3 : Gain  Gain=[0 1]  Multiplication=Matrix(K*u)
  Mux2 : Mux  Inputs=2
  Product2 : Product
  Product3 : Product
  Product7 : Product  Inputs=3
  Product8 : Product
  Product9 : Product  Inputs=3
  v_dq : Outport  VectorParamsAs1DForOutWhenUnconnected=off
  wires:
  Product3/1 -> Add7/2
  Product9/1 -> Add7/1
  Gain2/1 -> Product9/2
  om/1 -> Product9/3, Product7/3, Product3/1
  Product8/1 -> Product3/2
  Phif/1 -> Product8/2
  Product7/1 -> Gain1/1
  Gain3/1 -> Product7/2
  Product2/1 -> Product7/1, Product9/1
  L/1 -> Product2/1
  p/1 -> Product2/2, Product8/1
  Gain1/1 -> Mux2/1
  idq/1 -> Gain3/1, Gain2/1
  Add6/1 -> v_dq/1
  udq/1 -> Add6/1
  Add7/1 -> Mux2/2
  Mux2/1 -> Add6/2

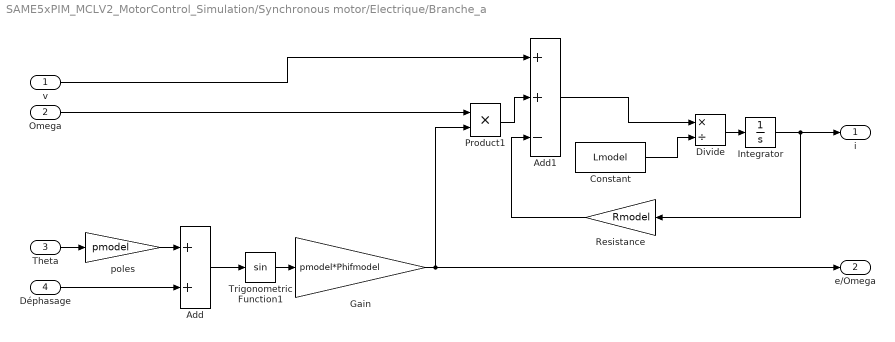
== system SAME5xPIM_MCLV2_MotorControl_Simulation/Synchronous motor/Electrique/Branche_a ==
  v : Inport
  Omega : Inport  Port=2
  Theta : Inport  Port=3
  Déphasage : Inport  Port=4
  Add : Sum
  Add1 : Sum  Inputs=++-
  Constant : Constant  Value=Lmodel
  Divide : Product  Inputs=*/
  Gain : Gain  Gain=pmodel*Phifmodel
  Integrator : Integrator
  Product1 : Product
  Resistance : Gain  Gain=Rmodel
  Trigonometric Function1 : Trigonometry
  poles : Gain  Gain=pmodel
  i : Outport  VectorParamsAs1DForOutWhenUnconnected=off
  e/Omega : Outport  Port=2  VectorParamsAs1DForOutWhenUnconnected=off
  wires:
  Divide/1 -> Integrator/1
  Resistance/1 -> Add1/3
  Product1/1 -> Add1/2
  Omega/1 -> Product1/1
  Trigonometric Function1/1 -> Gain/1
  Add1/1 -> Divide/1
  Integrator/1 -> Resistance/1, i/1
  Gain/1 -> Product1/2, e/Omega/1
  v/1 -> Add1/1
  Déphasage/1 -> Add/2
  poles/1 -> Add/1
  Theta/1 -> poles/1
  Add/1 -> Trigonometric Function1/1
  Constant/1 -> Divide/2

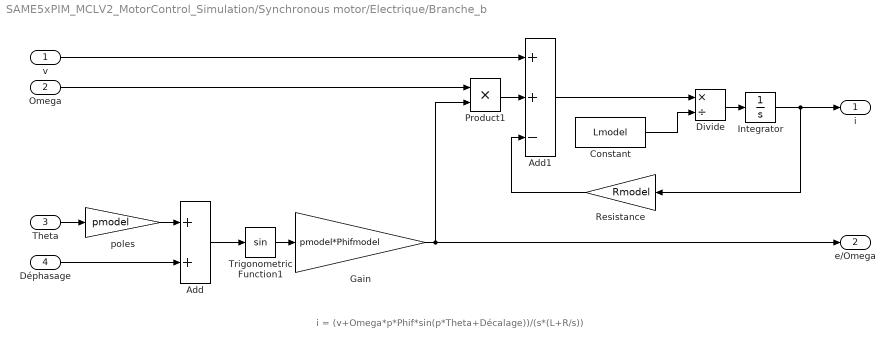
== system SAME5xPIM_MCLV2_MotorControl_Simulation/Synchronous motor/Electrique/Branche_b ==
  note: i = (v+Omega*p*Phif*sin(p*Theta+Décalage))/(s*(L+R/s))
  v : Inport
  Omega : Inport  Port=2
  Theta : Inport  Port=3
  Déphasage : Inport  Port=4
  Add : Sum
  Add1 : Sum  Inputs=++-
  Constant : Constant  Value=Lmodel
  Divide : Product  Inputs=*/
  Gain : Gain  Gain=pmodel*Phifmodel
  Integrator : Integrator
  Product1 : Product
  Resistance : Gain  Gain=Rmodel
  Trigonometric Function1 : Trigonometry
  poles : Gain  Gain=pmodel
  i : Outport  VectorParamsAs1DForOutWhenUnconnected=off
  e/Omega : Outport  Port=2  VectorParamsAs1DForOutWhenUnconnected=off
  wires:
  Divide/1 -> Integrator/1
  Resistance/1 -> Add1/3
  Product1/1 -> Add1/2
  Omega/1 -> Product1/1
  Trigonometric Function1/1 -> Gain/1
  Add1/1 -> Divide/1
  Integrator/1 -> Resistance/1, i/1
  Gain/1 -> Product1/2, e/Omega/1
  v/1 -> Add1/1
  Déphasage/1 -> Add/2
  poles/1 -> Add/1
  Theta/1 -> poles/1
  Add/1 -> Trigonometric Function1/1
  Constant/1 -> Divide/2

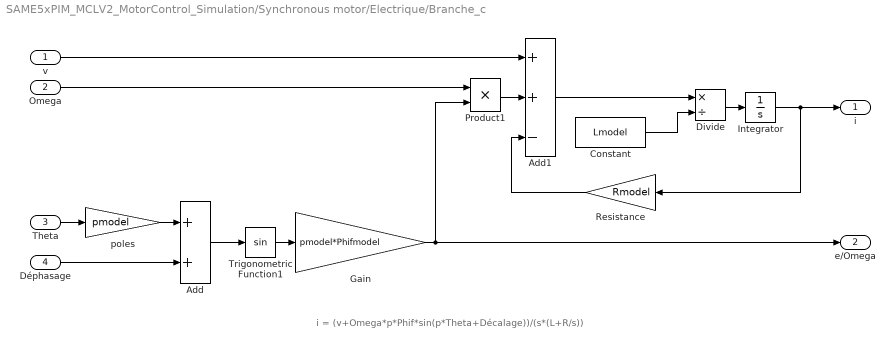
== system SAME5xPIM_MCLV2_MotorControl_Simulation/Synchronous motor/Electrique/Branche_c ==
  note: i = (v+Omega*p*Phif*sin(p*Theta+Décalage))/(s*(L+R/s))
  v : Inport
  Omega : Inport  Port=2
  Theta : Inport  Port=3
  Déphasage : Inport  Port=4
  Add : Sum
  Add1 : Sum  Inputs=++-
  Constant : Constant  Value=Lmodel
  Divide : Product  Inputs=*/
  Gain : Gain  Gain=pmodel*Phifmodel
  Integrator : Integrator
  Product1 : Product
  Resistance : Gain  Gain=Rmodel
  Trigonometric Function1 : Trigonometry
  poles : Gain  Gain=pmodel
  i : Outport  VectorParamsAs1DForOutWhenUnconnected=off
  e/Omega : Outport  Port=2  VectorParamsAs1DForOutWhenUnconnected=off
  wires:
  Divide/1 -> Integrator/1
  Resistance/1 -> Add1/3
  Product1/1 -> Add1/2
  Omega/1 -> Product1/1
  Trigonometric Function1/1 -> Gain/1
  Add1/1 -> Divide/1
  Integrator/1 -> Resistance/1, i/1
  Gain/1 -> Product1/2, e/Omega/1
  v/1 -> Add1/1
  Déphasage/1 -> Add/2
  poles/1 -> Add/1
  Theta/1 -> poles/1
  Add/1 -> Trigonometric Function1/1
  Constant/1 -> Divide/2

== system SAME5xPIM_MCLV2_MotorControl_Simulation/Control/Mechnical Control/Augmented state feedback/Clamping circuit ==
  note: The clamping enable or disable the integral action.
  Saturation : Inport  DisableCoverage=on
  preIntegrator : Inport  DisableCoverage=on  Port=2
  Compare To Zero1 : simulink/Logic and Bit Operations/Compare To Zero  relop=<=  OutDataTypeStr=boolean
  Delay : Delay  DelayLength=1  InitialCondition=0
  Multiply : Product
  Clamp : Outport  DisableCoverage=on  VectorParamsAs1DForOutWhenUnconnected=off
  wires:
  Delay/1 -> Multiply/1
  Saturation/1 -> Delay/1
  Multiply/1 -> Compare To Zero1/1
  preIntegrator/1 -> Multiply/2
  Compare To Zero1/1 -> Clamp/1

== system SAME5xPIM_MCLV2_MotorControl_Simulation/Control/Mechnical Control/Augmented state feedback/Integrator ==
  In1 : Inport
  Enable : EnablePort
  Discrete-Time Integrator : DiscreteIntegrator  SampleTime=1e-4  OutDataTypeStr=single  SaturateOnIntegerOverflow=on  ICPrevOutput=DiscIntNeverNeededParam  ICPrevScaledInput=DiscIntNeverNeededParam
  Out1 : Outport  VectorParamsAs1DForOutWhenUnconnected=off
  wires:
  In1/1 -> Discrete-Time Integrator/1
  Discrete-Time Integrator/1 -> Out1/1

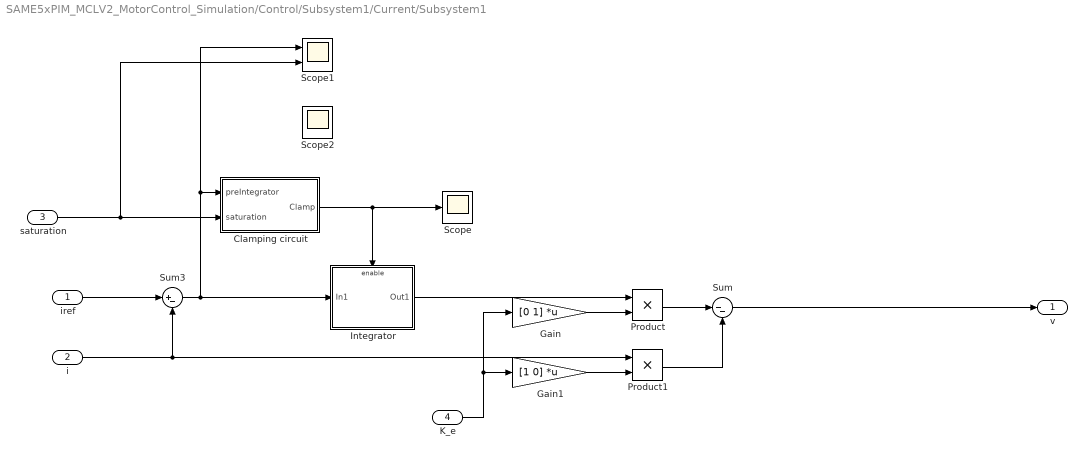
== system SAME5xPIM_MCLV2_MotorControl_Simulation/Control/Subsystem1/Current/Subsystem1 ==
  iref : Inport
  i : Inport  Port=2
  saturation : Inport  Port=3
  K_e : Inport  Port=4
  Clamping circuit : Subsystem
  Gain : Gain  Gain=[0 1]  Multiplication=Matrix(K*u)
  Gain1 : Gain  Gain=[1 0]  Multiplication=Matrix(K*u)
  Integrator : Subsystem
  Product : Product
  Product1 : Product
  Scope : Scope
  Scope1 : Scope  NumInputPorts=2
  Scope2 : Scope
  Sum : Sum  Inputs=|--  OutDataTypeStr=single  SaturateOnIntegerOverflow=on
  Sum3 : Sum  Inputs=|+-
  v : Outport  VectorParamsAs1DForOutWhenUnconnected=off
  wires:
  Sum/1 -> v/1
  Integrator/1(Out1) -> Product/1
  Clamping circuit/1(Clamp) -> Scope/1, Integrator/Enable
  iref/1 -> Sum3/1
  Sum3/1 -> Integrator/1(In1), Scope1/1, Clamping circuit/1(preIntegrator)
  i/1 -> Sum3/2, Product1/1
  Product/1 -> Sum/1
  Product1/1 -> Sum/2
  K_e/1 -> Gain/1, Gain1/1
  Gain/1 -> Product/2
  Gain1/1 -> Product1/2
  saturation/1 -> Scope1/2, Clamping circuit/2(saturation)

== system SAME5xPIM_MCLV2_MotorControl_Simulation/Control/Subsystem1/Current/Subsystem2 ==
  iref : Inport
  i : Inport  Port=2
  saturation : Inport  Port=3
  K_e : Inport  Port=4
  Clamping circuit : Subsystem
  Gain : Gain  Gain=[0 1]  Multiplication=Matrix(K*u)
  Gain1 : Gain  Gain=[1 0]  Multiplication=Matrix(K*u)
  Integrator : Subsystem
  Product : Product
  Product1 : Product
  Scope : Scope
  Sum : Sum  Inputs=|--  OutDataTypeStr=single  SaturateOnIntegerOverflow=on
  Sum3 : Sum  Inputs=|+-
  v : Outport  VectorParamsAs1DForOutWhenUnconnected=off
  wires:
  saturation/1 -> Clamping circuit/2(saturation)
  Gain1/1 -> Product1/2
  Gain/1 -> Product/2
  K_e/1 -> Gain1/1, Gain/1
  Product1/1 -> Sum/2
  Product/1 -> Sum/1
  i/1 -> Product1/1, Sum3/2
  Sum3/1 -> Clamping circuit/1(preIntegrator), Integrator/1(In1)
  iref/1 -> Sum3/1
  Clamping circuit/1(Clamp) -> Integrator/Enable
  Integrator/1(Out1) -> Product/1
  Sum/1 -> Scope/1, v/1

== system SAME5xPIM_MCLV2_MotorControl_Simulation/Control/Subsystem1/Voltage Saturation/Norm L2 ==
  In1 : Inport
  Dot Product : DotProduct  InputSameDT=on  OutDataTypeStr=Inherit: Inherit via internal rule
  Sqrt : Sqrt  SaturateOnIntegerOverflow=on
  y : Outport
  wires:
  In1/1 -> Dot Product/1, Dot Product/2
  Dot Product/1 -> Sqrt/1
  Sqrt/1 -> y/1

== system SAME5xPIM_MCLV2_MotorControl_Simulation/Control/Subsystem1/Current/Subsystem1/Clamping circuit ==
  note: The clamping enable or disable the integral action.
  preIntegrator : Inport  DisableCoverage=on
  saturation : Inport  DisableCoverage=on  Port=2
  Compare To Zero1 : simulink/Logic and Bit Operations/Compare To Zero  relop=<=  OutDataTypeStr=boolean
  Multiply : Product
  Clamp : Outport  DisableCoverage=on  VectorParamsAs1DForOutWhenUnconnected=off
  wires:
  saturation/1 -> Multiply/1
  Compare To Zero1/1 -> Clamp/1
  Multiply/1 -> Compare To Zero1/1
  preIntegrator/1 -> Multiply/2

== system SAME5xPIM_MCLV2_MotorControl_Simulation/Control/Subsystem1/Current/Subsystem1/Integrator ==
  In1 : Inport
  Enable : EnablePort
  Discrete-Time Integrator : DiscreteIntegrator  SampleTime=1e-4  OutDataTypeStr=single  ICPrevOutput=DiscIntNeverNeededParam  ICPrevScaledInput=DiscIntNeverNeededParam
  Out1 : Outport  VectorParamsAs1DForOutWhenUnconnected=off
  wires:
  Discrete-Time Integrator/1 -> Out1/1
  In1/1 -> Discrete-Time Integrator/1

== system SAME5xPIM_MCLV2_MotorControl_Simulation/Control/Subsystem1/Current/Subsystem2/Clamping circuit ==
  note: The clamping enable or disable the integral action.
  preIntegrator : Inport  DisableCoverage=on
  saturation : Inport  DisableCoverage=on  Port=2
  Compare To Zero1 : simulink/Logic and Bit Operations/Compare To Zero  relop=<=  OutDataTypeStr=boolean
  Multiply : Product
  Clamp : Outport  DisableCoverage=on  VectorParamsAs1DForOutWhenUnconnected=off
  wires:
  preIntegrator/1 -> Multiply/2
  Multiply/1 -> Compare To Zero1/1
  Compare To Zero1/1 -> Clamp/1
  saturation/1 -> Multiply/1

== system SAME5xPIM_MCLV2_MotorControl_Simulation/Control/Subsystem1/Current/Subsystem2/Integrator ==
  In1 : Inport
  Enable : EnablePort
  Discrete-Time Integrator : DiscreteIntegrator  SampleTime=1e-4  OutDataTypeStr=single  ICPrevOutput=DiscIntNeverNeededParam  ICPrevScaledInput=DiscIntNeverNeededParam
  Out1 : Outport  VectorParamsAs1DForOutWhenUnconnected=off
  wires:
  In1/1 -> Discrete-Time Integrator/1
  Discrete-Time Integrator/1 -> Out1/1
